simulink model "z_dummy"  (R2019a)
settings: Solver=VariableStepAuto  StartTime=0.0  StopTime=10.0  RelTol=1e-3
undefined symbols (not defined in the file or in its folder): Wind
settings Model: Creator=VTOL_HYD  LastModifiedBy=VTOL_HYD

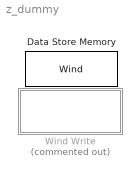
== system z_dummy ==
  Data Store Memory : DataStoreMemory  DataStoreName=Wind  ReadBeforeWriteMsg=warning  WriteAfterWriteMsg=warning  WriteAfterReadMsg=warning  InitialValue=[0;0;0;0;0;0;0;0;0;0]  ShowAdditionalParam=off
  Wind Write : Subsystem  Commented=on

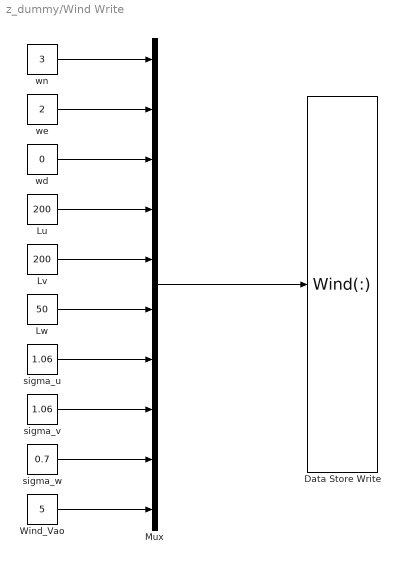
== system z_dummy/Wind Write ==
  Data Store Write : DataStoreWrite  DataStoreName=Wind  DataStoreElements=Wind(:)
  Lu : Constant  Value=200
  Lv : Constant  Value=200
  Lw : Constant  Value=50
  Mux : Mux  Inputs=10
  Wind_Vao : Constant  Value=5
  sigma_u : Constant  Value=1.06
  sigma_v : Constant  Value=1.06
  sigma_w : Constant  Value=0.7
  wd : Constant  Value=0
  "we " : Constant  Value=2
  "wn " : Constant  Value=3
  wires:
  Mux/1 -> Data Store Write/1
  "wn "/1 -> Mux/1
  "we "/1 -> Mux/2
  wd/1 -> Mux/3
  Lu/1 -> Mux/4
  Lv/1 -> Mux/5
  Lw/1 -> Mux/6
  sigma_u/1 -> Mux/7
  sigma_v/1 -> Mux/8
  sigma_w/1 -> Mux/9
  Wind_Vao/1 -> Mux/10
